simulink model "AdaptiveControl"  (R2022b)
settings: Solver=VariableStepAuto  StartTime=0.0  StopTime=10.0  RelTol=1e-3
undefined symbols (not defined in the file): a, fd1, fd2, g, k, p1, p2, p3, Td1, Td2
settings Model: Creator=Noor Hakam  LastModifiedBy=Noor Hakam

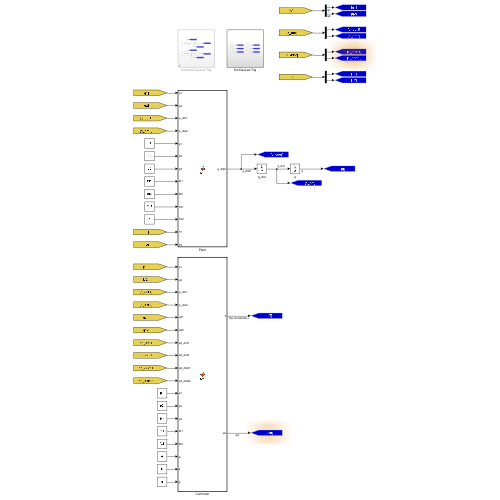
[thumbnail: Simulink's stored preview of the top-level diagram]
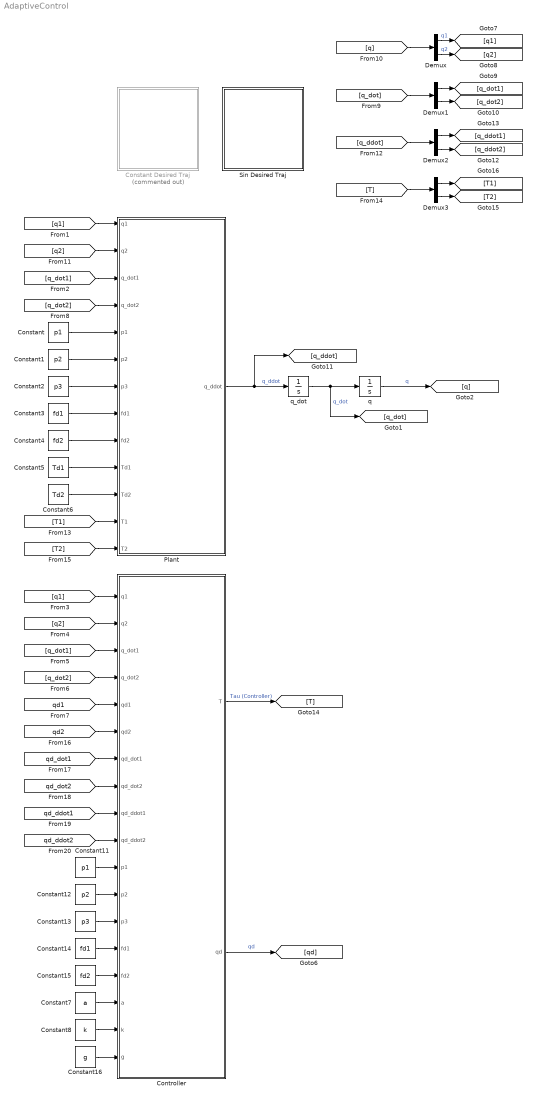
== system AdaptiveControl ==
  Constant : Constant  Value=p1
  Constant Desired Traj : Subsystem  Commented=on
  Constant1 : Constant  Value=p2
  Constant11 : Constant  Value=p1
  Constant12 : Constant  Value=p2
  Constant13 : Constant  Value=p3
  Constant14 : Constant  Value=fd1
  Constant15 : Constant  Value=fd2
  Constant16 : Constant  Value=g
  Constant2 : Constant  Value=p3
  Constant3 : Constant  Value=fd1
  Constant4 : Constant  Value=fd2
  Constant5 : Constant  Value=Td1
  Constant6 : Constant  Value=Td2
  Constant7 : Constant  Value=a
  Constant8 : Constant  Value=k
  Controller : MATLAB Function  TreatAsAtomicUnit=on
  Demux{,1..3} (4 alike) : Demux  Outputs=2
  Plant : MATLAB Function  TreatAsAtomicUnit=on
  Sin Desired Traj : Subsystem
  q : Integrator
  q_dot : Integrator
  wires:
  Constant13/1 -> Controller/13(p3)
  Demux1/1 -> [q_dot1]
  [q_dot] -> Demux1/1
  Demux/1 -> [q1]  "q1"
  [q_ddot] -> Demux2/1
  [qd_dot2] -> Controller/8(qd_dot2)
  [q_dot2] -> Controller/4(q_dot2)
  Demux/2 -> [q2]  "q2"
  [qd_ddot1] -> Controller/9(qd_ddot1)
  Constant11/1 -> Controller/11(p1)
  Constant12/1 -> Controller/12(p2)
  Demux1/2 -> [q_dot2]
  Controller/1(T) -> [T]  "Tau (Controller)"
  [q2] -> Plant/2(q2)
  [T2] -> Plant/13(T2)
  [q_dot2] -> Plant/4(q_dot2)
  [qd2] -> Controller/6(qd2)
  Demux2/2 -> [q_ddot2]
  Demux3/2 -> [T2]
  Demux3/1 -> [T1]
  [q1] -> Controller/1(q1)
  Constant6/1 -> Plant/11(Td2)
  [qd_dot1] -> Controller/7(qd_dot1)
  Constant7/1 -> Controller/16(a)
  Constant8/1 -> Controller/17(k)
  Constant5/1 -> Plant/10(Td1)
  [T] -> Demux3/1
  Controller/2(qd) -> [qd]  "qd"
  Constant/1 -> Plant/5(p1)
  Constant1/1 -> Plant/6(p2)
  Demux2/1 -> [q_ddot1]
  [q1] -> Plant/1(q1)
  Constant2/1 -> Plant/7(p3)
  Constant4/1 -> Plant/9(fd2)
  q_dot/1 -> q/1, [q_dot]  "q_dot"
  [qd_ddot2] -> Controller/10(qd_ddot2)
  Constant15/1 -> Controller/15(fd2)
  [T1] -> Plant/12(T1)
  Constant14/1 -> Controller/14(fd1)
  [q_dot1] -> Controller/3(q_dot1)
  q/1 -> [q]  "q"
  [q_dot1] -> Plant/3(q_dot1)
  Constant3/1 -> Plant/8(fd1)
  [qd1] -> Controller/5(qd1)
  Plant/1(q_ddot) -> q_dot/1, [q_ddot]  "q_ddot"
  [q2] -> Controller/2(q2)
  [q] -> Demux/1
  Constant16/1 -> Controller/18(g)

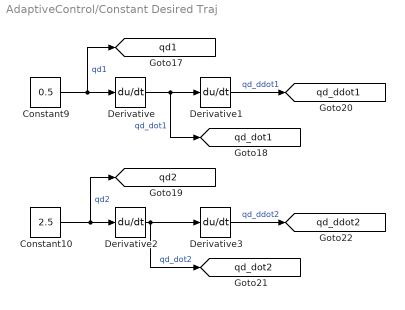
== system AdaptiveControl/Constant Desired Traj ==
  Constant10 : Constant  Value=2.5
  Constant9 : Constant  Value=0.5
  Derivative{,1..3} (4 alike) : Derivative
  tag scope: qd1=global, qd2=global, qd_ddot1=global, qd_ddot2=global, qd_dot1=global, qd_dot2=global
  wires:
  Constant9/1 -> Derivative/1, [qd1]  "qd1"
  Derivative2/1 -> Derivative3/1, [qd_dot2]  "qd_dot2"
  Derivative3/1 -> [qd_ddot2]  "qd_ddot2"
  Derivative1/1 -> [qd_ddot1]  "qd_ddot1"
  Constant10/1 -> Derivative2/1, [qd2]  "qd2"
  Derivative/1 -> Derivative1/1, [qd_dot1]  "qd_dot1"

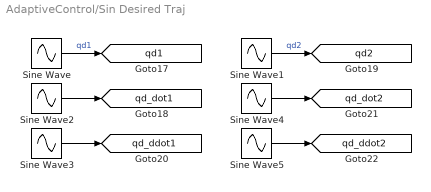
== system AdaptiveControl/Sin Desired Traj ==
  Sine Wave : Sin  Amplitude=0.5  SampleTime=0
  Sine Wave1 : Sin  Amplitude=2.5  Phase=pi / 2  SampleTime=0
  Sine Wave2 : Sin  Amplitude=0.5  Phase=pi / 2  SampleTime=0
  Sine Wave3 : Sin  Amplitude=-0.5  SampleTime=0
  Sine Wave4 : Sin  Amplitude=-5  SampleTime=0
  Sine Wave5 : Sin  Amplitude=-10  Phase=pi / 2  SampleTime=0
  tag scope: qd1=global, qd2=global, qd_ddot1=global, qd_ddot2=global, qd_dot1=global, qd_dot2=global
  wires:
  Sine Wave/1 -> [qd1]  "qd1"
  Sine Wave1/1 -> [qd2]  "qd2"
  Sine Wave2/1 -> [qd_dot1]
  Sine Wave3/1 -> [qd_ddot1]
  Sine Wave4/1 -> [qd_dot2]
  Sine Wave5/1 -> [qd_ddot2]

== matlab function AdaptiveControl/Plant ==
  data: q1 input; q_ddot output; q2 input; q_dot1 input; q_dot2 input; p1 input; p2 input; p3 input; fd1 input; fd2 input; Td1 input; Td2 input; T1 input; T2 input
function q_ddot   = fcn(q1, q2, q_dot1, q_dot2, p1, p2, p3, fd1, fd2, Td1, Td2, T1, T2)

%% Initialize
q_ddot = zeros(2, 1);
M = zeros(2, 2);
Vm = zeros(2, 2);
Fd = zeros(2, 2);
Td = zeros(2, 1);

q = [q1; q2];
q_dot = [q_dot1; q_dot2];
T = [T1; T2];

%% System parameters
M = [(p1 + (2 * p3 * cos(q(2))))       (p2 + (p3 * cos(q(2))));
     (p2 + (p3 * cos(q(2))))           (p2)];
Vm = [(-1 * p3 * sin(q(2)) * q_dot(2)) (-1 * p3 * sin(q(2)) * (q_dot(1) + q_dot(2)));
      (p3 * sin(q(2)) * q_dot(1))      (0)];
Fd = [fd1 0;
      0   fd2];
Td = [Td1; Td2];

%% System dynamics
invM = inv(M);
q_ddot = (invM * T) - (invM * (Vm * q_dot)) - (invM * (Fd * q_dot)) - Td;

== matlab function AdaptiveControl/Controller ==
  data: q1 input; T output; q2 input; q_dot1 input; q_dot2 input; qd1 input; qd2 input; qd_dot1 input; qd_dot2 input; qd_ddot1 input; qd_ddot2 input; p1 input; p2 input; p3 input; fd1 input; fd2 input; qd output; a input; k input; g input
function [T, qd] = fcn(q1, q2, q_dot1, q_dot2, qd1, qd2, qd_dot1,  qd_dot2, qd_ddot1, qd_ddot2, p1, p2, p3, fd1, fd2, a, k, g)

%% Initiatize
T = zeros(2, 1);
q = [q1; q2];
q_dot = [q_dot1; q_dot2];

%% System parameters
M = [(p1 + (2 * p3 * cos(q(2))))       (p2 + (p3 * cos(q(2))));
     (p2 + (p3 * cos(q(2))))           (p2)];
Vm = [(-1 * p3 * sin(q(2)) * q_dot(2)) (-1 * p3 * sin(q(2)) * (q_dot(1) + q_dot(2)));
      (p3 * sin(q(2)) * q_dot(1))      (0)];
Fd = [fd1 0;
      0   fd2];

%% Control gains
% a
% k
% g

%% Desired trajectory
qd = [qd1; qd2];
qd_dot = [qd_dot1; qd_dot2];
qd_ddot = [qd_ddot1; qd_ddot2];

%% Error system and auxillary signal
e = qd - q;
e_dot = qd_dot - q_dot;

r = e_dot + (a * e);

%% AC
Y1 = [qd_ddot(1) + a * e_dot(1); 0];
Y2 = [qd_ddot(2) +  a * e_dot(2); qd_ddot(1) + qd_ddot(2) + a * e_dot(1) + a * e_dot(2)];
Y3 = [-1 * sin(q(2)) * q_dot(2)^2 - 2 * q_dot(1) * sin(q(2)) * q_dot(2) + 2 * qd_ddot(1) * cos(q(2)) + qd_ddot(2) * cos(q(2)) + 2 * a * e_dot(1) * cos(q(2)) + a * e_dot(2) *cos(q(2)); sin(q(2)) * q_dot(1)^2 + qd_ddot(1) * cos(q(2)) + a * e_dot(1) * cos(q(2))];
Y4 = [q_dot(1); 0];
Y5 = [0; q_dot(2)];
Y = cat(2, Y1, Y2, Y3, Y4, Y5);

gamma = g * eye(5);
theta_hat = inv(gamma) * Y' * r;

T = (k * r) + (Y * theta_hat);
